simulink subsystem "WareHouseTaskRobotArchitecture"  (R2024b)
settings: Solver=VariableStepAuto  StartTime=0.0  StopTime=10.0  RelTol=1e-3
libraries: robotalgslib x1
settings Model: Creator=marcob  LastModifiedBy=mbecker

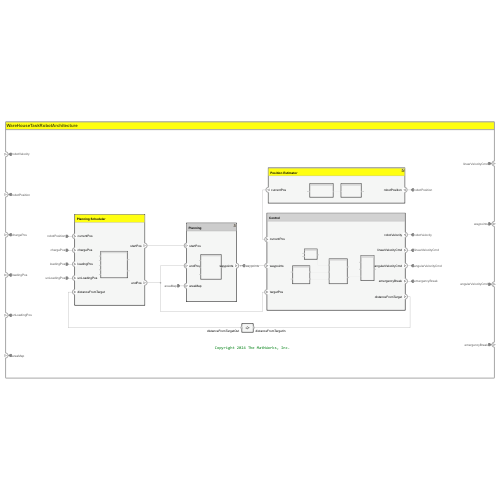
[thumbnail: Simulink's stored preview of the top-level diagram]
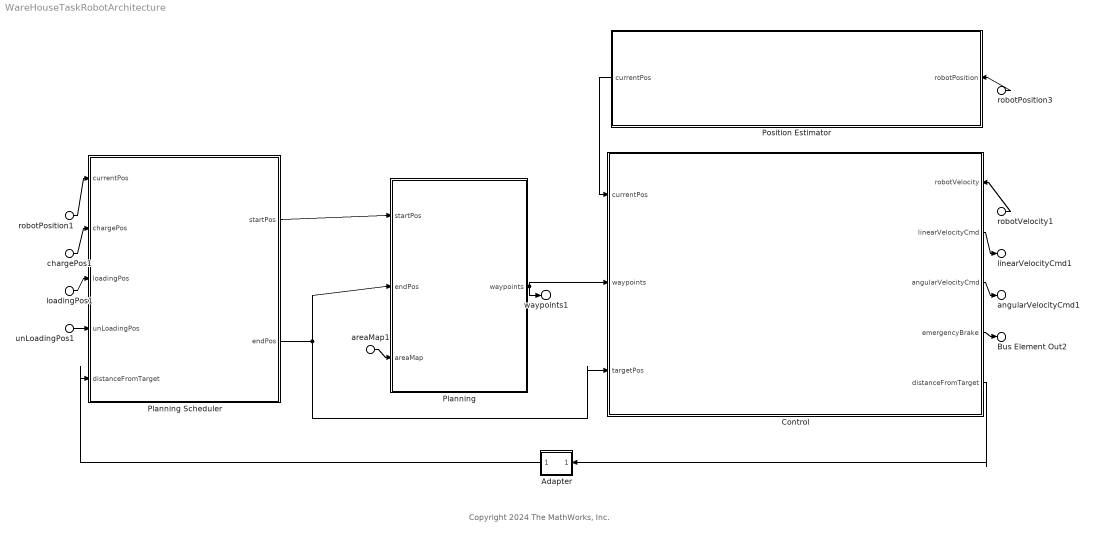
== system WareHouseTaskRobotArchitecture ==
  note: Copyright 2024 The MathWorks, Inc.
  robotVelocity1 : Inport  PortName=robotVelocity
  robotPosition1 : Inport  Port=2  PortName=robotPosition
  robotPosition3 : Inport  Port=2  PortName=robotPosition
  chargePos1 : Inport  Port=3  PortName=chargePos
  loadingPos1 : Inport  Port=4  PortName=loadingPos
  unLoadingPos1 : Inport  Port=5  PortName=unLoadingPos
  areaMap1 : Inport  Port=6  PortName=areaMap
  Adapter : Subsystem
      settings: PortSchema="{\"entries\":[{\"content\":{\"margin\":10,\"minimumSpacing\":15,\"sides\":[{\"content\":{\"connectorIds\":[\"Out1\"]},\"type\":\"ConnectorPlacement.EquallySpacedRectSide\",\"uuid\":\"fee8ae93-d3af-4af3-aba8-8bbb6c49b1e5\"},{\"content\":{\"connectorIds\":[\"In1\"],\"side\":\"RIGHT\"},\"type\":\"ConnectorPlacement.EquallySpacedRectSide\",\"uuid\":\"b0456245-7dcd-4816-a6fb-4f2f475968b2\"},{\"content\":{\"side\":\"TOP\"},\"type\":\"ConnectorPlacement.EquallySpacedRectSide\",\"uuid\":\"a975d676-5342-48fd-ad94-ed1438dae107\"},{\"content\":{\"side\":\"BOTTOM\"},\"type\":\"ConnectorPlacement.EquallySpacedRectSide\",\"uuid\":\"ae62e64a-8a9f-4616-a235-281c09bea0dd\"}]},\"type\":\"ConnectorPlacement.EquallySpacedConnector\",\"uuid\":\"79662a43-5fa9-4b9c-9165-dcb3e1feed12\"}],\"packageUris\":[\"http://schema.mathworks.com/mf0/Connector/R2020b\"],\"version\":\"1.0\"}"
  Control : Subsystem
      settings: PortSchema="{\"entries\":[{\"content\":{\"headerSize\":26,\"margin\":15,\"minimumSpacing\":25,\"sides\":[{\"content\":{\"connectorIds\":[\"In2\",\"In4\",\"In3\"]},\"type\":\"ConnectorPlacement.EquallySpacedRectSide\",\"uuid\":\"f08cfdbd-fecc-40c8-9b37-8f1ddd10c25d\"},{\"content\":{\"connectorIds\":[\"In1\",\"Out1\",\"Out2\",\"Out3\",\"Out4\"],\"side\":\"RIGHT\"},\"type\":\"ConnectorPlacement.EquallySpacedRectSide\",\"uuid\":\"23957699-09ca-40e0-a43c-3ce051c3f904\"},{\"content\":{\"side\":\"TOP\"},\"type\":\"ConnectorPlacement.EquallySpacedRectSide\",\"uuid\":\"fa22ca7b-887e-4d4d-86f4-92b1b6513fc8\"}]},\"type\":\"ConnectorPlacement.EquallySpacedConnector\",\"uuid\":\"b2ceef94-ae2e-48b1-8273-16d9e5f01224\"}],\"packageUris\":[\"http://schema.mathworks.com/mf0/Connector/R2020b\"],\"version\":\"1.0\"}"
  Planning : Subsystem
      settings: PortSchema="{\"entries\":[{\"content\":{\"headerSize\":26,\"margin\":15,\"minimumSpacing\":25,\"sides\":[{\"content\":{\"connectorIds\":[\"In1\",\"In2\",\"In3\"]},\"type\":\"ConnectorPlacement.EquallySpacedRectSide\",\"uuid\":\"f08cfdbd-fecc-40c8-9b37-8f1ddd10c25d\"},{\"content\":{\"connectorIds\":[\"Out1\"],\"side\":\"RIGHT\"},\"type\":\"ConnectorPlacement.EquallySpacedRectSide\",\"uuid\":\"23957699-09ca-40e0-a43c-3ce051c3f904\"},{\"content\":{\"side\":\"TOP\"},\"type\":\"ConnectorPlacement.EquallySpacedRectSide\",\"uuid\":\"fa22ca7b-887e-4d4d-86f4-92b1b6513fc8\"}]},\"type\":\"ConnectorPlacement.EquallySpacedConnector\",\"uuid\":\"b2ceef94-ae2e-48b1-8273-16d9e5f01224\"}],\"packageUris\":[\"http://schema.mathworks.com/mf0/Connector/R2020b\"],\"version\":\"1.0\"}"
  Planning Scheduler : Subsystem
      settings: PortSchema="{\"entries\":[{\"content\":{\"headerSize\":26,\"margin\":15,\"minimumSpacing\":25,\"sides\":[{\"content\":{\"connectorIds\":[\"In1\",\"In2\",\"In3\",\"In4\",\"In5\"]},\"type\":\"ConnectorPlacement.EquallySpacedRectSide\",\"uuid\":\"f08cfdbd-fecc-40c8-9b37-8f1ddd10c25d\"},{\"content\":{\"connectorIds\":[\"Out1\",\"Out2\"],\"side\":\"RIGHT\"},\"type\":\"ConnectorPlacement.EquallySpacedRectSide\",\"uuid\":\"23957699-09ca-40e0-a43c-3ce051c3f904\"},{\"content\":{\"side\":\"TOP\"},\"type\":\"ConnectorPlacement.EquallySpacedRectSide\",\"uuid\":\"fa22ca7b-887e-4d4d-86f4-92b1b6513fc8\"}]},\"type\":\"ConnectorPlacement.EquallySpacedConnector\",\"uuid\":\"b2ceef94-ae2e-48b1-8273-16d9e5f01224\"}],\"packageUris\":[\"http://schema.mathworks.com/mf0/Connector/R2020b\"],\"version\":\"1.0\"}"
  Position Estimator : Subsystem
      settings: PortSchema="{\"entries\":[{\"content\":{\"headerSize\":26,\"margin\":15,\"minimumSpacing\":25,\"sides\":[{\"content\":{\"connectorIds\":[\"Out1\"]},\"type\":\"ConnectorPlacement.EquallySpacedRectSide\",\"uuid\":\"fee8ae93-d3af-4af3-aba8-8bbb6c49b1e5\"},{\"content\":{\"connectorIds\":[\"In1\"],\"side\":\"RIGHT\"},\"type\":\"ConnectorPlacement.EquallySpacedRectSide\",\"uuid\":\"b0456245-7dcd-4816-a6fb-4f2f475968b2\"},{\"content\":{\"side\":\"TOP\"},\"type\":\"ConnectorPlacement.EquallySpacedRectSide\",\"uuid\":\"a975d676-5342-48fd-ad94-ed1438dae107\"}]},\"type\":\"ConnectorPlacement.EquallySpacedConnector\",\"uuid\":\"79662a43-5fa9-4b9c-9165-dcb3e1feed12\"}],\"packageUris\":[\"http://schema.mathworks.com/mf0/Connector/R2020b\"],\"version\":\"1.0\"}"
  linearVelocityCmd1 : Outport  PortName=linearVelocityCmd
  Bus Element Out2 : Outport  Port=2  PortName=emergencyBrake
  waypoints1 : Outport  Port=3  PortName=waypoints
  angularVelocityCmd1 : Outport  Port=4  PortName=angularVelocityCmd
  wires:
  Planning Scheduler/2(endPos) -> Planning/2(endPos), Control/3(targetPos)
  robotPosition1/1 -> Planning Scheduler/1(currentPos)
  Planning Scheduler/1(startPos) -> Planning/1(startPos)
  Control/2(angularVelocityCmd) -> angularVelocityCmd1/1
  Planning/1(waypoints) -> Control/4(waypoints), waypoints1/1
  unLoadingPos1/1 -> Planning Scheduler/4(unLoadingPos)
  chargePos1/1 -> Planning Scheduler/2(chargePos)
  loadingPos1/1 -> Planning Scheduler/3(loadingPos)
  areaMap1/1 -> Planning/3(areaMap)
  Control/1(linearVelocityCmd) -> linearVelocityCmd1/1
  Adapter/1(distanceFromTargetOut) -> Planning Scheduler/5(distanceFromTarget)
  Control/4(distanceFromTarget) -> Adapter/1(distanceFromTargetIn)
  robotPosition3/1 -> Position Estimator/1(robotPosition)
  Position Estimator/1(currentPos) -> Control/2(currentPos)
  Control/3(emergencyBrake) -> Bus Element Out2/1
  robotVelocity1/1 -> Control/1(robotVelocity)

== system WareHouseTaskRobotArchitecture/Adapter ==
  In Bus Element : Inport  PortName=distanceFromTargetIn
  Out Bus Element : Outport  PortName=distanceFromTargetOut
  wires:
  In Bus Element/1 -> Out Bus Element/1

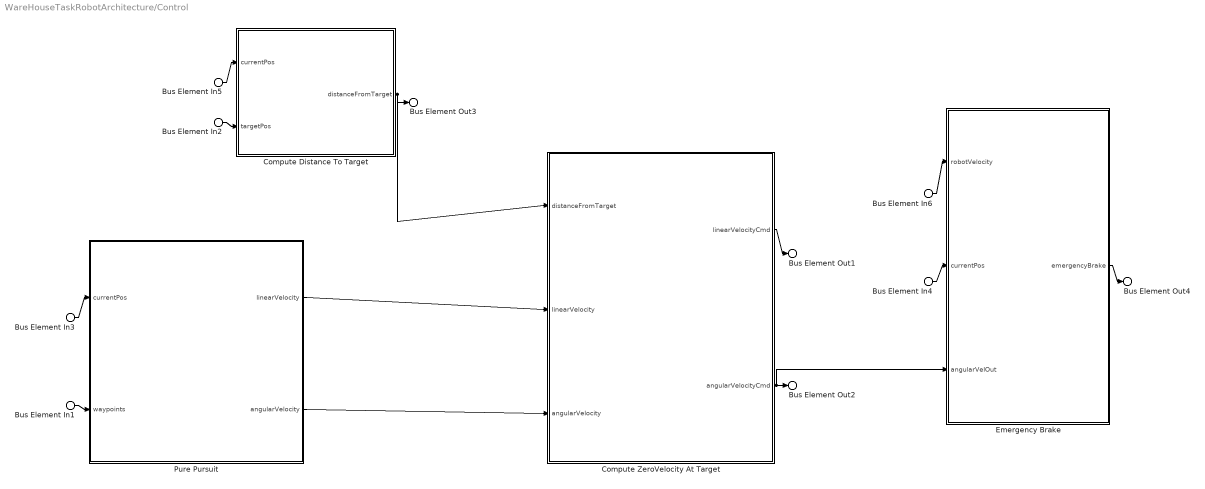
== system WareHouseTaskRobotArchitecture/Control ==
  Bus Element In6 : Inport  PortName=robotVelocity
  Bus Element In3 : Inport  Port=2  PortName=currentPos
  Bus Element In5 : Inport  Port=2  PortName=currentPos
  Bus Element In4 : Inport  Port=2  PortName=currentPos
  Bus Element In2 : Inport  Port=3  PortName=targetPos
  Bus Element In1 : Inport  Port=4  PortName=waypoints
  Compute Distance To Target : Subsystem
      settings: PortSchema="{\"entries\":[{\"content\":{\"headerSize\":26,\"margin\":15,\"minimumSpacing\":25,\"sides\":[{\"content\":{\"connectorIds\":[\"In1\",\"In2\"]},\"type\":\"ConnectorPlacement.EquallySpacedRectSide\",\"uuid\":\"f08cfdbd-fecc-40c8-9b37-8f1ddd10c25d\"},{\"content\":{\"connectorIds\":[\"Out1\"],\"side\":\"RIGHT\"},\"type\":\"ConnectorPlacement.EquallySpacedRectSide\",\"uuid\":\"23957699-09ca-40e0-a43c-3ce051c3f904\"},{\"content\":{\"side\":\"TOP\"},\"type\":\"ConnectorPlacement.EquallySpacedRectSide\",\"uuid\":\"fa22ca7b-887e-4d4d-86f4-92b1b6513fc8\"}]},\"type\":\"ConnectorPlacement.EquallySpacedConnector\",\"uuid\":\"b2ceef94-ae2e-48b1-8273-16d9e5f01224\"}],\"packageUris\":[\"http://schema.mathworks.com/mf0/Connector/R2020b\"],\"version\":\"1.0\"}"
  Compute ZeroVelocity At Target : Subsystem
      settings: PortSchema="{\"entries\":[{\"content\":{\"headerSize\":26,\"margin\":15,\"minimumSpacing\":25,\"sides\":[{\"content\":{\"connectorIds\":[\"In1\",\"In2\",\"In3\"]},\"type\":\"ConnectorPlacement.EquallySpacedRectSide\",\"uuid\":\"f08cfdbd-fecc-40c8-9b37-8f1ddd10c25d\"},{\"content\":{\"connectorIds\":[\"Out1\",\"Out2\"],\"side\":\"RIGHT\"},\"type\":\"ConnectorPlacement.EquallySpacedRectSide\",\"uuid\":\"23957699-09ca-40e0-a43c-3ce051c3f904\"},{\"content\":{\"side\":\"TOP\"},\"type\":\"ConnectorPlacement.EquallySpacedRectSide\",\"uuid\":\"fa22ca7b-887e-4d4d-86f4-92b1b6513fc8\"}]},\"type\":\"ConnectorPlacement.EquallySpacedConnector\",\"uuid\":\"b2ceef94-ae2e-48b1-8273-16d9e5f01224\"}],\"packageUris\":[\"http://schema.mathworks.com/mf0/Connector/R2020b\"],\"version\":\"1.0\"}"
  Emergency Brake : Subsystem  Variant=on  VariantControlMode=label  VariantControl=Emergency Break  LabelModeActiveChoice=Emergency Brake Active
      settings: PortSchema="{\"entries\":[{\"content\":{\"headerSize\":38,\"margin\":15,\"minimumSpacing\":25,\"sides\":[{\"content\":{\"connectorIds\":[\"In1\",\"In2\",\"In3\"]},\"type\":\"ConnectorPlacement.EquallySpacedRectSide\",\"uuid\":\"f08cfdbd-fecc-40c8-9b37-8f1ddd10c25d\"},{\"content\":{\"connectorIds\":[\"Out1\"],\"side\":\"RIGHT\"},\"type\":\"ConnectorPlacement.EquallySpacedRectSide\",\"uuid\":\"23957699-09ca-40e0-a43c-3ce051c3f904\"},{\"content\":{\"side\":\"TOP\"},\"type\":\"ConnectorPlacement.EquallySpacedRectSide\",\"uuid\":\"fa22ca7b-887e-4d4d-86f4-92b1b6513fc8\"}]},\"type\":\"ConnectorPlacement.EquallySpacedConnector\",\"uuid\":\"b2ceef94-ae2e-48b1-8273-16d9e5f01224\"}],\"packageUris\":[\"http://schema.mathworks.com/mf0/Connector/R2020b\"],\"version\":\"1.0\"}"
  Pure Pursuit : Subsystem
      settings: PortSchema="{\"entries\":[{\"content\":{\"headerSize\":26,\"margin\":15,\"minimumSpacing\":25,\"sides\":[{\"content\":{\"connectorIds\":[\"In1\",\"In2\"]},\"type\":\"ConnectorPlacement.EquallySpacedRectSide\",\"uuid\":\"f08cfdbd-fecc-40c8-9b37-8f1ddd10c25d\"},{\"content\":{\"connectorIds\":[\"Out1\",\"Out2\"],\"side\":\"RIGHT\"},\"type\":\"ConnectorPlacement.EquallySpacedRectSide\",\"uuid\":\"23957699-09ca-40e0-a43c-3ce051c3f904\"},{\"content\":{\"side\":\"TOP\"},\"type\":\"ConnectorPlacement.EquallySpacedRectSide\",\"uuid\":\"fa22ca7b-887e-4d4d-86f4-92b1b6513fc8\"}]},\"type\":\"ConnectorPlacement.EquallySpacedConnector\",\"uuid\":\"b2ceef94-ae2e-48b1-8273-16d9e5f01224\"}],\"packageUris\":[\"http://schema.mathworks.com/mf0/Connector/R2020b\"],\"version\":\"1.0\"}"
  Bus Element Out1 : Outport  PortName=linearVelocityCmd
  Bus Element Out2 : Outport  Port=2  PortName=angularVelocityCmd
  Bus Element Out4 : Outport  Port=3  PortName=emergencyBrake
  Bus Element Out3 : Outport  Port=4  PortName=distanceFromTarget
  wires:
  Emergency Brake/1(emergencyBrake) -> Bus Element Out4/1
  Bus Element In4/1 -> Emergency Brake/2(currentPos)
  Bus Element In6/1 -> Emergency Brake/1(robotVelocity)
  Compute ZeroVelocity At Target/2(angularVelocityCmd) -> Emergency Brake/3(angularVelOut), Bus Element Out2/1
  Compute ZeroVelocity At Target/1(linearVelocityCmd) -> Bus Element Out1/1
  Pure Pursuit/1(linearVelocity) -> Compute ZeroVelocity At Target/2(linearVelocity)
  Pure Pursuit/2(angularVelocity) -> Compute ZeroVelocity At Target/3(angularVelocity)
  Compute Distance To Target/1(distanceFromTarget) -> Compute ZeroVelocity At Target/1(distanceFromTarget), Bus Element Out3/1
  Bus Element In2/1 -> Compute Distance To Target/2(targetPos)
  Bus Element In5/1 -> Compute Distance To Target/1(currentPos)
  Bus Element In1/1 -> Pure Pursuit/2(waypoints)
  Bus Element In3/1 -> Pure Pursuit/1(currentPos)

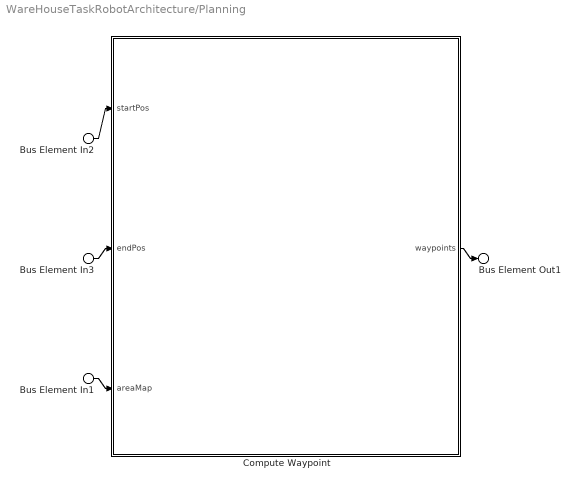
== system WareHouseTaskRobotArchitecture/Planning ==
  Bus Element In2 : Inport  PortName=startPos
  Bus Element In3 : Inport  Port=2  PortName=endPos
  Bus Element In1 : Inport  Port=3  PortName=areaMap
  Compute Waypoint : Subsystem
      settings: PortSchema="{\"entries\":[{\"content\":{\"headerSize\":26,\"margin\":15,\"minimumSpacing\":25,\"sides\":[{\"content\":{\"connectorIds\":[\"In1\",\"In2\",\"In3\"]},\"type\":\"ConnectorPlacement.EquallySpacedRectSide\",\"uuid\":\"f08cfdbd-fecc-40c8-9b37-8f1ddd10c25d\"},{\"content\":{\"connectorIds\":[\"Out1\"],\"side\":\"RIGHT\"},\"type\":\"ConnectorPlacement.EquallySpacedRectSide\",\"uuid\":\"23957699-09ca-40e0-a43c-3ce051c3f904\"},{\"content\":{\"side\":\"TOP\"},\"type\":\"ConnectorPlacement.EquallySpacedRectSide\",\"uuid\":\"fa22ca7b-887e-4d4d-86f4-92b1b6513fc8\"}]},\"type\":\"ConnectorPlacement.EquallySpacedConnector\",\"uuid\":\"b2ceef94-ae2e-48b1-8273-16d9e5f01224\"}],\"packageUris\":[\"http://schema.mathworks.com/mf0/Connector/R2020b\"],\"version\":\"1.0\"}"
  Bus Element Out1 : Outport  PortName=waypoints
  wires:
  Compute Waypoint/1(waypoints) -> Bus Element Out1/1
  Bus Element In2/1 -> Compute Waypoint/1(startPos)
  Bus Element In3/1 -> Compute Waypoint/2(endPos)
  Bus Element In1/1 -> Compute Waypoint/3(areaMap)

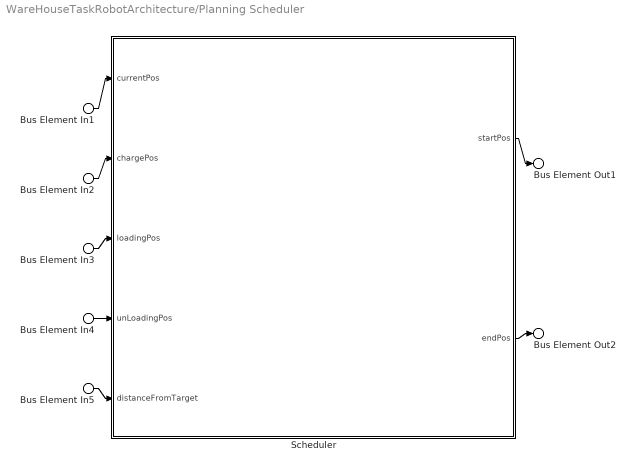
== system WareHouseTaskRobotArchitecture/Planning Scheduler ==
  Bus Element In1 : Inport  PortName=currentPos
  Bus Element In2 : Inport  Port=2  PortName=chargePos
  Bus Element In3 : Inport  Port=3  PortName=loadingPos
  Bus Element In4 : Inport  Port=4  PortName=unLoadingPos
  Bus Element In5 : Inport  Port=5  PortName=distanceFromTarget
  Scheduler : Subsystem
      settings: PortSchema="{\"entries\":[{\"content\":{\"headerSize\":26,\"margin\":15,\"minimumSpacing\":25,\"sides\":[{\"content\":{\"connectorIds\":[\"In1\",\"In2\",\"In3\",\"In4\",\"In5\"]},\"type\":\"ConnectorPlacement.EquallySpacedRectSide\",\"uuid\":\"fee8ae93-d3af-4af3-aba8-8bbb6c49b1e5\"},{\"content\":{\"connectorIds\":[\"Out1\",\"Out2\"],\"side\":\"RIGHT\"},\"type\":\"ConnectorPlacement.EquallySpacedRectSide\",\"uuid\":\"b0456245-7dcd-4816-a6fb-4f2f475968b2\"},{\"content\":{\"side\":\"TOP\"},\"type\":\"ConnectorPlacement.EquallySpacedRectSide\",\"uuid\":\"a975d676-5342-48fd-ad94-ed1438dae107\"}]},\"type\":\"ConnectorPlacement.EquallySpacedConnector\",\"uuid\":\"79662a43-5fa9-4b9c-9165-dcb3e1feed12\"}],\"packageUris\":[\"http://schema.mathworks.com/mf0/Connector/R2020b\"],\"version\":\"1.0\"}"
  Bus Element Out1 : Outport  PortName=startPos
  Bus Element Out2 : Outport  Port=2  PortName=endPos
  wires:
  Scheduler/1(startPos) -> Bus Element Out1/1
  Scheduler/2(endPos) -> Bus Element Out2/1
  Bus Element In4/1 -> Scheduler/4(unLoadingPos)
  Bus Element In3/1 -> Scheduler/3(loadingPos)
  Bus Element In5/1 -> Scheduler/5(distanceFromTarget)
  Bus Element In1/1 -> Scheduler/1(currentPos)
  Bus Element In2/1 -> Scheduler/2(chargePos)

== system WareHouseTaskRobotArchitecture/Position Estimator ==
  Bus Element In1 : Inport  PortName=robotPosition
  Processing And Filtering : Subsystem
      settings: PortSchema="{\"entries\":[{\"content\":{\"headerSize\":26,\"margin\":15,\"minimumSpacing\":25,\"sides\":[{\"content\":{\"connectorIds\":[\"Out1\"]},\"type\":\"ConnectorPlacement.EquallySpacedRectSide\",\"uuid\":\"fee8ae93-d3af-4af3-aba8-8bbb6c49b1e5\"},{\"content\":{\"connectorIds\":[\"In1\"],\"side\":\"RIGHT\"},\"type\":\"ConnectorPlacement.EquallySpacedRectSide\",\"uuid\":\"b0456245-7dcd-4816-a6fb-4f2f475968b2\"},{\"content\":{\"side\":\"TOP\"},\"type\":\"ConnectorPlacement.EquallySpacedRectSide\",\"uuid\":\"a975d676-5342-48fd-ad94-ed1438dae107\"}]},\"type\":\"ConnectorPlacement.EquallySpacedConnector\",\"uuid\":\"79662a43-5fa9-4b9c-9165-dcb3e1feed12\"}],\"packageUris\":[\"http://schema.mathworks.com/mf0/Connector/R2020b\"],\"version\":\"1.0\"}"
  Unit Conversion : Subsystem
      settings: PortSchema="{\"entries\":[{\"content\":{\"headerSize\":26,\"margin\":15,\"minimumSpacing\":25,\"sides\":[{\"content\":{\"connectorIds\":[\"Out1\"]},\"type\":\"ConnectorPlacement.EquallySpacedRectSide\",\"uuid\":\"fee8ae93-d3af-4af3-aba8-8bbb6c49b1e5\"},{\"content\":{\"connectorIds\":[\"In1\"],\"side\":\"RIGHT\"},\"type\":\"ConnectorPlacement.EquallySpacedRectSide\",\"uuid\":\"b0456245-7dcd-4816-a6fb-4f2f475968b2\"},{\"content\":{\"side\":\"TOP\"},\"type\":\"ConnectorPlacement.EquallySpacedRectSide\",\"uuid\":\"a975d676-5342-48fd-ad94-ed1438dae107\"}]},\"type\":\"ConnectorPlacement.EquallySpacedConnector\",\"uuid\":\"79662a43-5fa9-4b9c-9165-dcb3e1feed12\"}],\"packageUris\":[\"http://schema.mathworks.com/mf0/Connector/R2020b\"],\"version\":\"1.0\"}"
  Bus Element Out1 : Outport  PortName=currentPos
  wires:
  Processing And Filtering/1(currentPos) -> Bus Element Out1/1
  Unit Conversion/1(pos_eng_unit) -> Processing And Filtering/1(pos_eng_unit)
  Bus Element In1/1 -> Unit Conversion/1(robotPosition)

== system WareHouseTaskRobotArchitecture/Control/Compute Distance To Target ==
  Bus Element In2 : Inport  PortName=currentPos
  Bus Element In1 : Inport  Port=2  PortName=targetPos
  Check Distance To Goal : Subsystem
  Bus Element Out1 : Outport  PortName=distanceFromTarget
  wires:
  Bus Element In2/1 -> Check Distance To Goal/2(currentPose)
  Bus Element In1/1 -> Check Distance To Goal/1(robotGoal)
  Check Distance To Goal/1(atGoal) -> Bus Element Out1/1

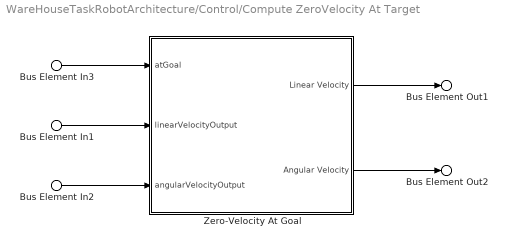
== system WareHouseTaskRobotArchitecture/Control/Compute ZeroVelocity At Target ==
  Bus Element In3 : Inport  PortName=distanceFromTarget
  Bus Element In1 : Inport  Port=2  PortName=linearVelocity
  Bus Element In2 : Inport  Port=3  PortName=angularVelocity
  Zero-Velocity At Goal : Subsystem
  Bus Element Out1 : Outport  PortName=linearVelocityCmd
  Bus Element Out2 : Outport  Port=2  PortName=angularVelocityCmd
  wires:
  Zero-Velocity At Goal/2(Angular Velocity) -> Bus Element Out2/1
  Zero-Velocity At Goal/1(Linear Velocity) -> Bus Element Out1/1
  Bus Element In2/1 -> Zero-Velocity At Goal/3(angularVelocityOutput)
  Bus Element In1/1 -> Zero-Velocity At Goal/2(linearVelocityOutput)
  Bus Element In3/1 -> Zero-Velocity At Goal/1(atGoal)

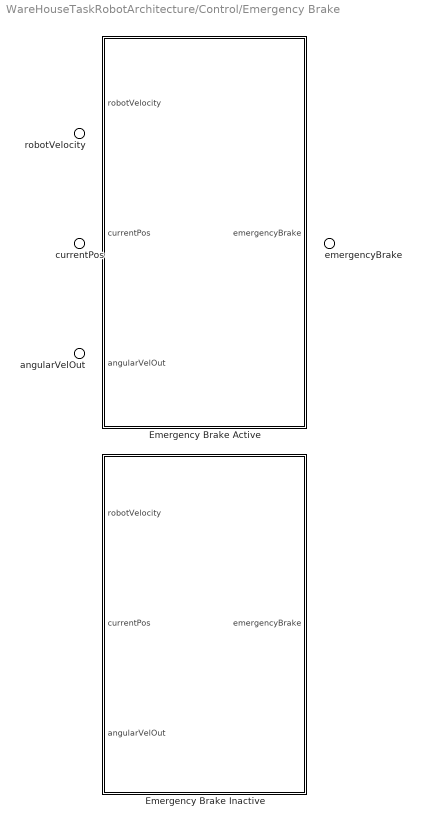
== system WareHouseTaskRobotArchitecture/Control/Emergency Brake ==
  robotVelocity : Inport
  currentPos : Inport  Port=2
  angularVelOut : Inport  Port=3
  Emergency Brake Active : Subsystem  VariantControl=Emergency Brake Active
      settings: PortSchema="{\"entries\":[{\"content\":{\"headerSize\":26,\"margin\":15,\"minimumSpacing\":25,\"sides\":[{\"content\":{\"connectorIds\":[\"In1\",\"In2\",\"In3\"]},\"type\":\"ConnectorPlacement.EquallySpacedRectSide\",\"uuid\":\"f08cfdbd-fecc-40c8-9b37-8f1ddd10c25d\"},{\"content\":{\"connectorIds\":[\"Out1\"],\"side\":\"RIGHT\"},\"type\":\"ConnectorPlacement.EquallySpacedRectSide\",\"uuid\":\"23957699-09ca-40e0-a43c-3ce051c3f904\"},{\"content\":{\"side\":\"TOP\"},\"type\":\"ConnectorPlacement.EquallySpacedRectSide\",\"uuid\":\"fa22ca7b-887e-4d4d-86f4-92b1b6513fc8\"}]},\"type\":\"ConnectorPlacement.EquallySpacedConnector\",\"uuid\":\"b2ceef94-ae2e-48b1-8273-16d9e5f01224\"}],\"packageUris\":[\"http://schema.mathworks.com/mf0/Connector/R2020b\"],\"version\":\"1.0\"}"
  Emergency Brake Inactive : Subsystem  VariantControl=Emergency Brake Inactive
      settings: PortSchema="{\"entries\":[{\"content\":{\"headerSize\":26,\"margin\":15,\"minimumSpacing\":25,\"sides\":[{\"content\":{\"connectorIds\":[\"In1\",\"In2\",\"In3\"]},\"type\":\"ConnectorPlacement.EquallySpacedRectSide\",\"uuid\":\"5ccff003-76f7-4779-807a-91871d9674a7\"},{\"content\":{\"connectorIds\":[\"Out1\"],\"side\":\"RIGHT\"},\"type\":\"ConnectorPlacement.EquallySpacedRectSide\",\"uuid\":\"6cd9e982-3620-451d-98aa-950993e654a7\"},{\"content\":{\"side\":\"TOP\"},\"type\":\"ConnectorPlacement.EquallySpacedRectSide\",\"uuid\":\"2bbc8775-e2c4-4cb5-b84c-c760113c580e\"}]},\"type\":\"ConnectorPlacement.EquallySpacedConnector\",\"uuid\":\"e16273e9-2f6a-4fc6-ae3c-1aa32184264a\"}],\"packageUris\":[\"http://schema.mathworks.com/mf0/Connector/R2020b\"],\"version\":\"1.0\"}"
  emergencyBrake : Outport

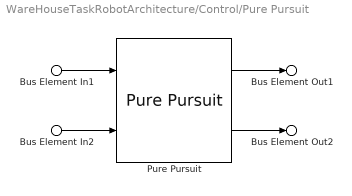
== system WareHouseTaskRobotArchitecture/Control/Pure Pursuit ==
  Bus Element In1 : Inport  PortName=currentPos
  Bus Element In2 : Inport  Port=2  PortName=waypoints
  Pure Pursuit : robotalgslib/Pure Pursuit  DesiredLinearVelocityPort=off  DesiredLinearVelocity=0.1  MaxAngularVelocity=1.0  LookaheadDistancePort=off  LookaheadDistance=0.5  TargetDirPort=off  SimulateUsing=Code generation
  Bus Element Out1 : Outport  PortName=linearVelocity
  Bus Element Out2 : Outport  Port=2  PortName=angularVelocity
  wires:
  Pure Pursuit/2 -> Bus Element Out2/1
  Pure Pursuit/1 -> Bus Element Out1/1
  Bus Element In2/1 -> Pure Pursuit/2
  Bus Element In1/1 -> Pure Pursuit/1

== system WareHouseTaskRobotArchitecture/Planning/Compute Waypoint ==
  Bus Element In1 : Inport  PortName=startPos
  Bus Element In2 : Inport  Port=2  PortName=endPos
  Bus Element In3 : Inport  Port=3  PortName=areaMap
  Planner : MATLAB Function  TreatAsAtomicUnit=on
  Bus Element Out1 : Outport  PortName=waypoints
  wires:
  Planner/1(waypoints) -> Bus Element Out1/1  "planOutput"
  Bus Element In3/1 -> Planner/3(mapMatrix)
  Bus Element In2/1 -> Planner/2(endPos)
  Bus Element In1/1 -> Planner/1(startPos)

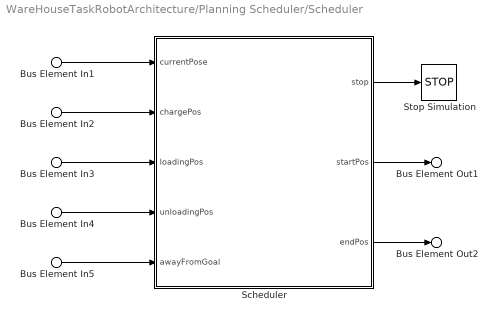
== system WareHouseTaskRobotArchitecture/Planning Scheduler/Scheduler ==
  Bus Element In1 : Inport  PortName=currentPos
  Bus Element In2 : Inport  Port=2  PortName=chargePos
  Bus Element In3 : Inport  Port=3  PortName=loadingPos
  Bus Element In4 : Inport  Port=4  PortName=unLoadingPos
  Bus Element In5 : Inport  Port=5  PortName=distanceFromTarget
  Scheduler : Stateflow chart  TreatAsAtomicUnit=on
  Stop Simulation : Stop
  Bus Element Out1 : Outport  PortName=startPos
  Bus Element Out2 : Outport  Port=2  PortName=endPos
  wires:
  Scheduler/2(startPos) -> Bus Element Out1/1
  Scheduler/3(endPos) -> Bus Element Out2/1
  Bus Element In4/1 -> Scheduler/4(unloadingPos)
  Bus Element In5/1 -> Scheduler/5(awayFromGoal)
  Bus Element In3/1 -> Scheduler/3(loadingPos)
  Bus Element In2/1 -> Scheduler/2(chargePos)
  Bus Element In1/1 -> Scheduler/1(currentPose)
  Scheduler/1(stop) -> Stop Simulation/1

== system WareHouseTaskRobotArchitecture/Position Estimator/Processing And Filtering ==
  Bus Element In1 : Inport  PortName=pos_eng_unit
  Bus Element Out1 : Outport  PortName=currentPos
  wires:
  Bus Element In1/1 -> Bus Element Out1/1

== system WareHouseTaskRobotArchitecture/Position Estimator/Unit Conversion ==
  Bus Element In1 : Inport  PortName=robotPosition
  Bus Element Out1 : Outport  PortName=pos_eng_unit
  wires:
  Bus Element In1/1 -> Bus Element Out1/1

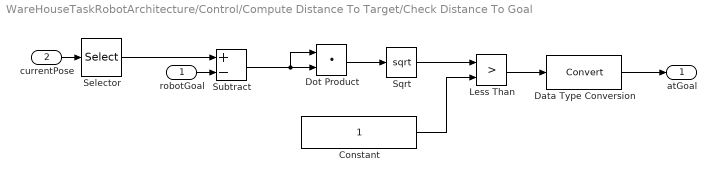
== system WareHouseTaskRobotArchitecture/Control/Compute Distance To Target/Check Distance To Goal ==
  robotGoal : Inport
  currentPose : Inport  Port=2
  Constant : Constant
  Data Type Conversion : DataTypeConversion  SampleTime=[0 1]  SaturateOnIntegerOverflow=off  RndMeth=Floor
  Dot Product : DotProduct  OutDataTypeStr=Inherit: Inherit via internal rule
  Less Than : RelationalOperator  Operator=>  OutDataTypeStr=boolean  RndMeth=Simplest  InputSameDT=off
  Selector : Selector  InputPortWidth=3  IndexOptions=Index vector (dialog)  Indices=[1 2]  OutputSizes=1
  Sqrt : Sqrt
  Subtract : Sum  Inputs=+-
  atGoal : Outport
  wires:
  Data Type Conversion/1 -> atGoal/1
  Selector/1 -> Subtract/1
  Subtract/1 -> Dot Product/2, Dot Product/1
  Sqrt/1 -> Less Than/1
  Less Than/1 -> Data Type Conversion/1
  currentPose/1 -> Selector/1
  Constant/1 -> Less Than/2
  Dot Product/1 -> Sqrt/1
  robotGoal/1 -> Subtract/2

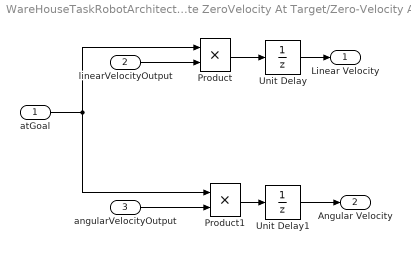
== system WareHouseTaskRobotArchitecture/Control/Compute ZeroVelocity At Target/Zero-Velocity At Goal ==
  atGoal : Inport
  linearVelocityOutput : Inport  Port=2
  angularVelocityOutput : Inport  Port=3
  Product : Product
  Product1 : Product
  Unit Delay : UnitDelay  SampleTime=-1  HasFrameUpgradeWarning=on
  Unit Delay1 : UnitDelay  SampleTime=-1  HasFrameUpgradeWarning=on
  Linear Velocity : Outport  OutDataTypeStr=double
  Angular Velocity : Outport  Port=2  OutDataTypeStr=double
  wires:
  Unit Delay1/1 -> Angular Velocity/1
  Unit Delay/1 -> Linear Velocity/1
  Product1/1 -> Unit Delay1/1
  Product/1 -> Unit Delay/1
  linearVelocityOutput/1 -> Product/2
  angularVelocityOutput/1 -> Product1/2
  atGoal/1 -> Product/1, Product1/1

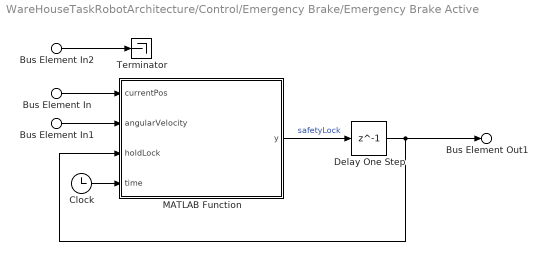
== system WareHouseTaskRobotArchitecture/Control/Emergency Brake/Emergency Brake Active ==
  Bus Element In2 : Inport  PortName=robotVelocity
  Bus Element In : Inport  Port=2  PortName=currentPos
  Bus Element In1 : Inport  Port=3  PortName=angularVelOut
  Clock : Clock
  Delay One Step : Delay  DelayLength=1
  MATLAB Function : MATLAB Function  TreatAsAtomicUnit=on
  Terminator : Terminator
  Bus Element Out1 : Outport  PortName=emergencyBrake
  wires:
  Bus Element In2/1 -> Terminator/1
  Bus Element In1/1 -> MATLAB Function/2(angularVelocity)
  Bus Element In/1 -> MATLAB Function/1(currentPos)
  Clock/1 -> MATLAB Function/4(time)
  Delay One Step/1 -> MATLAB Function/3(holdLock), Bus Element Out1/1
  MATLAB Function/1(y) -> Delay One Step/1  "safetyLock"

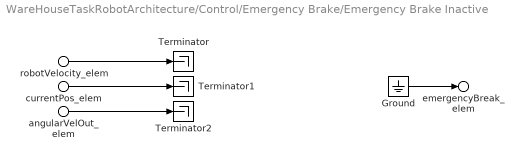
== system WareHouseTaskRobotArchitecture/Control/Emergency Brake/Emergency Brake Inactive ==
  robotVelocity_elem : Inport  PortName=robotVelocity
  currentPos_elem : Inport  Port=2  PortName=currentPos
  angularVelOut_elem : Inport  Port=3  PortName=angularVelOut
  Ground : Ground
  Terminator : Terminator
  Terminator1 : Terminator
  Terminator2 : Terminator
  emergencyBreak_elem : Outport  PortName=emergencyBrake
  wires:
  angularVelOut_elem/1 -> Terminator2/1
  currentPos_elem/1 -> Terminator1/1
  robotVelocity_elem/1 -> Terminator/1
  Ground/1 -> emergencyBreak_elem/1

== matlab function WareHouseTaskRobotArchitecture/Planning/Compute Waypoint/Planner ==
  settings: updateMethod=DISCRETE
  data: startPos input size=[1 2]; endPos input size=[1 2]; waypoints output size=[100 2]; mapMatrix input
function waypoints = planning(startPos, endPos, mapMatrix)

persistent waypointsInternal
persistent prevStartPos
persistent prevEndPos

% Set constant parameters
maxNumNodes = 100;

% Initialize persistent variables that are used downstream
if isempty(prevStartPos)
    prevStartPos = startPos;
end

if isempty(prevEndPos)
    prevEndPos = endPos;
end

isNewPath = (~isequal(prevStartPos, startPos) || ~isequal(prevEndPos, endPos));

if isempty(waypointsInternal) || isNewPath
    % Two conditions in which waypoints must be set: they are not yet
    % initialized, or they are initialized, but the current start and end
    % do not match those used to generate the previous set of waypoints
    [waypointsInternal] = planPath(mapMatrix, maxNumNodes, startPos, endPos);
end

% Update the outputs
waypoints = waypointsInternal;

% Update the persistent variables that indicate previous state
prevStartPos = startPos;
prevEndPos = endPos;

%% Helper Function

function wayPoints = planPath(mapMatrix, maxNodes, startPos, endPos)
    
    % Create a probabilistic roadmap
    map = binaryOccupancyMap(mapMatrix);
    prm = mobileRobotPRM(map, maxNodes);
    
    % Find a path between two points
    xy = findpath(prm, startPos(:)', endPos(:)');
    wayPoints = repmat(endPos(:)', maxNodes, 1);
    
    % Number of nodes that are actually used
    numNodes = length(xy);
    wayPoints(1:numNodes,:) = xy;    

end

end

== stateflow chart WareHouseTaskRobotArchitecture/Planning Scheduler/Scheduler/Scheduler ==
  settings: sampleTime=0.01
  state Unloading
    entry, during:
    endPos = unloadingPos';
  state Loading
    entry,during:
    endPos = loadingPos';
  state Charging
    entry, during:
    endPos = chargePos';
  (default) -> Loading : {startPos = chargePos';}
  Loading -> Unloading : [~awayFromGoal && after(stopDelay, tick)]
      |
      | {startPos = currentPose(1:2)';}
  Unloading -> Charging : [~awayFromGoal  && after(stopDelay, tick)]
      | {startPos = currentPose(1:2)';}
  Charging -> (junction 201) : [~awayFromGoal]{stop = 1;}
  data: currentPose input; stop output =0; chargePos input size=[2 1]; loadingPos input size=[2 1]; unloadingPos input size=[2 1]; startPos output size=[1, 2]; endPos output size=[1, 2]; awayFromGoal input; stopDelay local =0.7e4

== matlab function WareHouseTaskRobotArchitecture/Control/Emergency Brake/Emergency Brake Active/MATLAB Function ==
  settings: updateMethod=DISCRETE
  data: currentPos input; angularVelocity input; y output; holdLock input; time input
function y = safetyLock(currentPos, angularVelocity, holdLock, time)
    active = true;
    maxErrorAngle = 0.5;
    maxPredictionTime = 1;

    persistent previousAngle;
    persistent predictedAngle;
    persistent previousTime;
    persistent predictionTime;
    persistent previousAngularVelocity;

    if isempty(previousAngle) && time>0
        previousAngle = currentPos(3);
        previousTime = time;
        predictedAngle = currentPos(3);
        previousAngularVelocity = angularVelocity;
        predictionTime = 0;
        y=0;
        return;
    elseif isempty(previousAngle)
        y=0;
        return;
    end
    sampleTime = time - previousTime;
    predictionTime = predictionTime + sampleTime;
    previousTime = time;

    if(predictionTime>maxPredictionTime)
        predictionTime = 0;
        predictedAngle = currentPos(3);
    else    
        predictedAngle = previousAngle + previousAngularVelocity*sampleTime;
    end
    previousAngularVelocity = angularVelocity;
    previousAngle = predictedAngle;
    errorAngle = abs(angdiff(predictedAngle,currentPos(3)));
    if active && (holdLock || errorAngle>maxErrorAngle)
        y = 1;
    else
        y = 0;
    end
end
